simulink model "vehicle_cornering_aero_model"  (R2025b)
settings: Solver=VariableStepAuto  StartTime=0.0  StopTime=100  RelTol=1e-3
model workspace (MAT data in the model file):
  xdot_o = Simulink.Parameter
  xdot_o.Complexity = 'real'
  xdot_o.Dimensions = [1 1]
  xdot_o.DataType = 'auto'
undefined symbols (not defined in the file or in its folder): Ab, Af, brakeBias, cf, Cl, cr, Gamma, gearRatio, hg, Ixx, Kpf, Kpr, l, m, maxPower, maxRev, maxWhlAng, Prs, RCf, RCr, rho, SteerFrq, tireD, track, vref, wd
libraries: simulink_extras x4, simulink x3, vehdynlibtirecommon x3, sharedtransform x3, autolibutils x2, vehdynlibdriver x1, vehdynlibtire x1, autolibshared x1
(part 1 of 2)
settings Model: SimulationMode=accelerator  Creator=keisu  LastModifiedBy=keisu
settings DataIOCC: ReturnWorkspaceOutputs=off

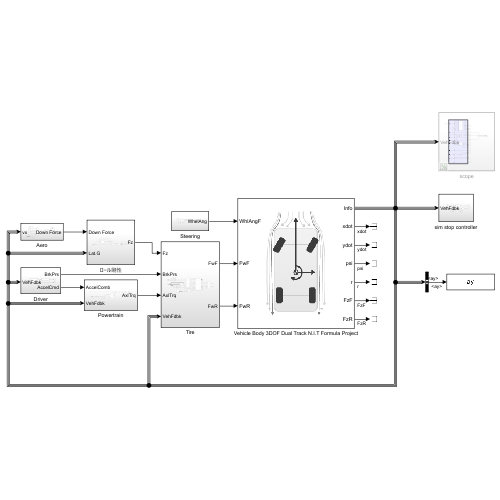
[thumbnail: Simulink's stored preview of the top-level diagram]
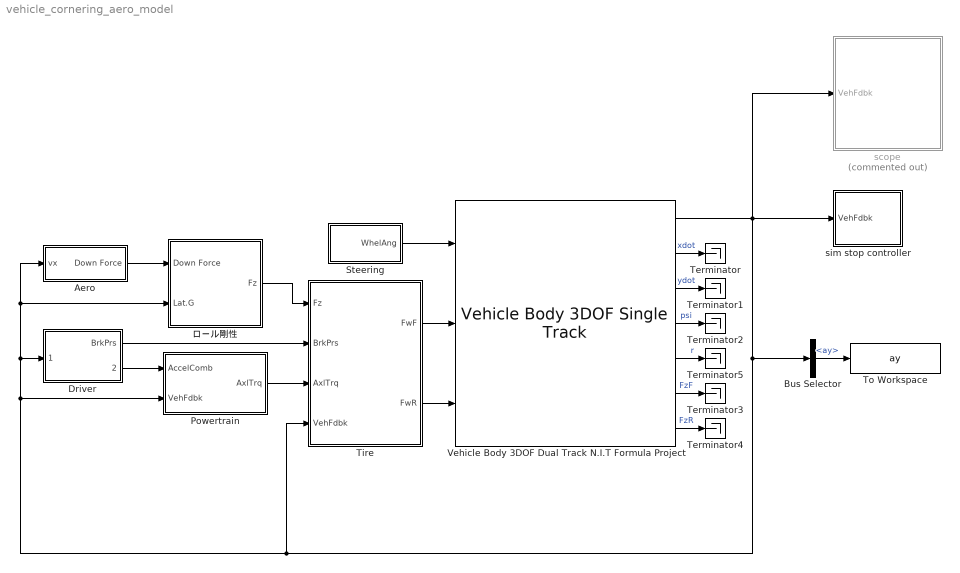
== system vehicle_cornering_aero_model ==
  Aero : Subsystem
  Bus Selector : BusSelector  OutputSignals=BdyFrm.Cg.Acc.ay
  Driver : Subsystem
  Powertrain : Subsystem
  Steering : Subsystem
  Terminator{,1..5} (6 alike) : Terminator
  Tire : Subsystem
  To Workspace : ToWorkspace  VariableName=ay  SaveFormat=Timeseries  SampleTime=-1
  Vehicle Body 3DOF Dual Track N.I.T Formula Project : autolibshared/Vehicle Body 3DOF Single Track  trackMode=Dual  inputMode=External forces  frontSteerMode=on  rearSteerMode=off  windMode=off  muMode=off  extFMode=off  extMMode=off  htchFMode=off  htchMMode=off  extXo=off  extpsio=off  extxdoto=off  extro=off  extYo=off  extTamb=off  extydoto=off  aMode=2  NF=2  NR=2  m=m  a=l*(1-wd)  b=l*wd  h=hg-0.0254*tireD/2  dh=1  hh=0.2  X_o=0  xdot_o=0  CalphaMode=off  sigmaMode=on  d=0  hl=0  w=track  Cy_f=12e3  Cy_r=11e3  sigma_f=.1  sigma_r=.1  alpha_f_brk=[-0.785, -0.628, -0.471, -0.314, -0.157, 0.000, 0.157, 0.314, 0.471, 0.628, 0.785]  Cy_f_data=[2000, 3000, 4000, 5500, 7000, 9000, 7000, 5500, 4000, 3000, 2000]  alpha_r_brk=[-0.785, -0.628, -0.471, -0.314, -0.157, 0.000, 0.157, 0.314, 0.471, 0.628, 0.785]  Cy_r_data=[2000, 3000, 4000, 5500, 7000, 9000, 7000, 5500, 4000, 3000, 2000]  Y_o=0  ydot_o=0  Izz=Izz  psi_o=0  r_o=0  Af=Af  Cd=Cd  Cl=Cl  Cpm=.1  beta_w=[0 0.01:0.01:0.3]  Cs=[0:0.03:0.9]  Cym=[0 1e-6:0.01:0.3]  Pabs=101325  Tair=AirTemp  g=9.81  mu=1  xdot_tol=.01  Fznom=5000  Fxtire_sat=7e4  Fytire_sat=7e4  longOff=0  latOff=0  vertOff=0  wrapAng=off
      settings: LibrarySourceBlock=vehdynlibeom/Vehicle Body 3DOF Dual Track
  scope : Subsystem  Commented=on
  sim stop controller : Subsystem
  ロール剛性 : Subsystem
  wires:
  Vehicle Body 3DOF Dual Track N.I.T Formula Project/1 -> sim stop controller/1(VehFdbk), scope/1(VehFdbk), Bus Selector/1, Aero/1(vx), ロール剛性/2(Lat.G), Driver/1(VehFdbk), Powertrain/2(VehFdbk), Tire/4(VehFdbk)
  Tire/1(FwF) -> Vehicle Body 3DOF Dual Track N.I.T Formula Project/2
  Tire/2(FwR) -> Vehicle Body 3DOF Dual Track N.I.T Formula Project/3
  Vehicle Body 3DOF Dual Track N.I.T Formula Project/2 -> Terminator/1  "xdot"
  Vehicle Body 3DOF Dual Track N.I.T Formula Project/3 -> Terminator1/1  "ydot"
  Vehicle Body 3DOF Dual Track N.I.T Formula Project/4 -> Terminator2/1  "psi"
  Vehicle Body 3DOF Dual Track N.I.T Formula Project/5 -> Terminator5/1  "r"
  Vehicle Body 3DOF Dual Track N.I.T Formula Project/6 -> Terminator3/1  "FzF"
  Vehicle Body 3DOF Dual Track N.I.T Formula Project/7 -> Terminator4/1  "FzR"
  Powertrain/1(AxlTrq) -> Tire/3(AxlTrq)
  ロール剛性/1(Fz) -> Tire/1(Fz)
  Driver/1(BrkPrs) -> Tire/2(BrkPrs)
  Driver/2(AccelCmd) -> Powertrain/1(AccelComb)
  Steering/1(WhelAng) -> Vehicle Body 3DOF Dual Track N.I.T Formula Project/1
  Bus Selector/1 -> To Workspace/1  "<ay>"
  Aero/1(Down Force) -> ロール剛性/1(Down Force)

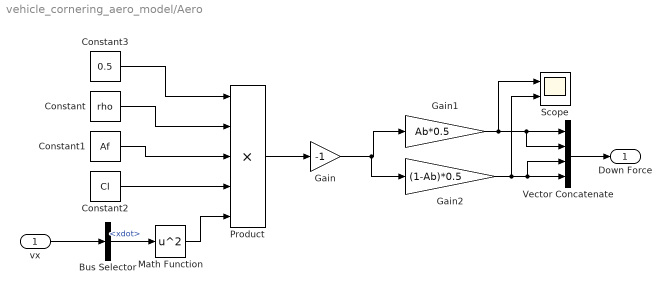
== system vehicle_cornering_aero_model/Aero ==
  vx : Inport
  Bus Selector : BusSelector  OutputSignals=BdyFrm.Cg.Vel.xdot
  Constant : Constant  Value=rho
  Constant1 : Constant  Value=Af
  Constant2 : Constant  Value=Cl
  Constant3 : Constant  Value=0.5
  Gain : Gain  Gain=-1
  Gain1 : Gain  Gain=Ab*0.5
  Gain2 : Gain  Gain=(1-Ab)*0.5
  Math Function : Math  Operator=square
  Product : Product  Inputs=5
  Scope : Scope  NumInputPorts=2
      settings: ActiveDisplayYMinimum=-1  ActiveDisplayYMaximum=1  DataLoggingVariableName=ScopeData2
  Vector Concatenate : Concatenate  NumInputs=4
  Down Force : Outport
  wires:
  vx/1 -> Bus Selector/1
  Constant3/1 -> Product/1
  Constant/1 -> Product/2
  Constant1/1 -> Product/3
  Constant2/1 -> Product/4
  Bus Selector/1 -> Math Function/1  "<xdot>"
  Math Function/1 -> Product/5
  Product/1 -> Gain/1
  Vector Concatenate/1 -> Down Force/1
  Gain/1 -> Gain2/1, Gain1/1
  Gain1/1 -> Scope/1, Vector Concatenate/2, Vector Concatenate/1
  Gain2/1 -> Vector Concatenate/4, Vector Concatenate/3, Scope/2

== system vehicle_cornering_aero_model/Driver ==
  VehFdbk : Inport
  Brake Hydraulics : Subsystem
  Driver : Subsystem
  BrkPrs : Outport
  AccelCmd : Outport  Port=2
  wires:
  Driver/1(DecelCmd) -> Brake Hydraulics/1(BrkPrsCmd)
  Driver/2(AccelCmd) -> AccelCmd/1
  Brake Hydraulics/1(BrkPrs) -> BrkPrs/1
  VehFdbk/1 -> Driver/1(VehFdbk)

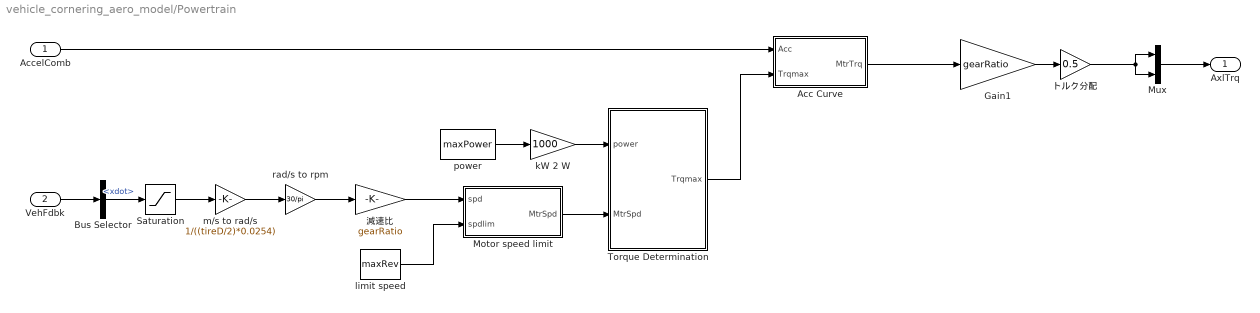
== system vehicle_cornering_aero_model/Powertrain ==
  AccelComb : Inport
  VehFdbk : Inport  Port=2
  Acc Curve : MATLAB Function  TreatAsAtomicUnit=on
  Bus Selector : BusSelector  OutputSignals=BdyFrm.Cg.Vel.xdot
  Gain1 : Gain  Gain=gearRatio
  Motor speed limit : MATLAB Function  TreatAsAtomicUnit=on
  Mux : Mux  Inputs=2
  Saturation : Saturate  UpperLimit=inf  LowerLimit=0
  Torque Determination : MATLAB Function  TreatAsAtomicUnit=on
  kW 2 W : Gain  Gain=1000
  limit speed : Constant  Value=maxRev
  m/s to rad/s : Gain  Gain=1/((tireD/2)*0.0254)
  power : Constant  Value=maxPower
  rad/s to rpm : Gain  Gain=30/pi
  トルク分配 : Gain  Gain=0.5
  減速比 : Gain  Gain=gearRatio
  AxlTrq : Outport
  wires:
  power/1 -> kW 2 W/1
  limit speed/1 -> Motor speed limit/2(spdlim)
  rad/s to rpm/1 -> 減速比/1
  Torque Determination/1(Trqmax) -> Acc Curve/2(Trqmax)
  AccelComb/1 -> Acc Curve/1(Acc)
  減速比/1 -> Motor speed limit/1(spd)
  m/s to rad/s/1 -> rad/s to rpm/1
  kW 2 W/1 -> Torque Determination/1(power)
  Motor speed limit/1(MtrSpd) -> Torque Determination/2(MtrSpd)
  Saturation/1 -> m/s to rad/s/1
  VehFdbk/1 -> Bus Selector/1
  Gain1/1 -> トルク分配/1
  Mux/1 -> AxlTrq/1
  Acc Curve/1(MtrTrq) -> Gain1/1
  Bus Selector/1 -> Saturation/1  "<xdot>"
  トルク分配/1 -> Mux/2, Mux/1

== system vehicle_cornering_aero_model/Steering ==
  <1 : Saturate  UpperLimit=1  LowerLimit=-1
  Degrees to Radians2 : simulink_extras/Transformations/Degrees to Radians
  Dot Product : DotProduct  OutDataTypeStr=Inherit: Inherit via internal rule
  Vector Concatenate : Concatenate
  最大ホール端転舵角 : Constant  Value=maxWhlAng
  転舵周波数 : simulink/Sources/Ramp  slope=1/SteerFrq  start=steerstartTime  InitialOutput=0
  WhelAng : Outport
  wires:
  転舵周波数/1 -> <1/1
  Dot Product/1 -> Degrees to Radians2/1
  <1/1 -> Dot Product/2
  最大ホール端転舵角/1 -> Dot Product/1
  Degrees to Radians2/1 -> Vector Concatenate/2, Vector Concatenate/1
  Vector Concatenate/1 -> WhelAng/1

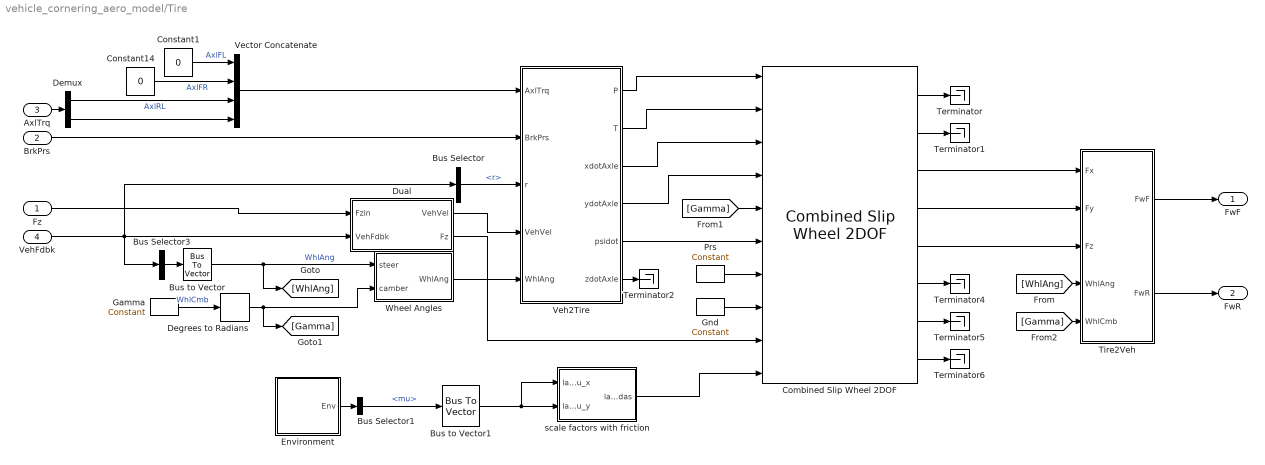
== system vehicle_cornering_aero_model/Tire ==
  Fz : Inport
  BrkPrs : Inport  Port=2
  AxlTrq : Inport  Port=3
  VehFdbk : Inport  Port=4
  Bus Selector : BusSelector  OutputSignals=BdyFrm.Cg.AngVel.r
  Bus Selector1 : BusSelector  OutputSignals=Gnd.mu
  Bus Selector3 : BusSelector  OutputSignals=BdyFrm.FrntAxl.Steer.WhlAngFL,BdyFrm.FrntAxl.Steer.WhlAngFR,BdyFrm.RearAxl.Steer.WhlAngRL,BdyFrm.RearAxl.Steer.WhlAngRR  OutputAsBus=on
  Bus to Vector : BusToVector
  Bus to Vector1 : BusToVector
  Combined Slip Wheel 2DOF : vehdynlibtire/Combined Slip Wheel 2DOF  tireType=External file  tireParamSet=TIRfile  vertType=Magic Formula  plySteer=off  turnslip=off  BrakeType=Disc  mu_static=mu_static  mu_kinetic=mu_kinetic  drum_abore=0.0508  drum_a=0.123  drum_c=0.212  drum_r=0.15  drum_theta1=0  drum_theta2=126  disk_abore=disk_abore  Rm=Rm  num_pads=num_pads  brake_p_bpt=[1 11.4736842105263 21.9473684210526 32.4210526315789 42.8947368421053 53.3684210526316 63.8421052631579 74.3157894736842 84.7894736842105 95.2631578947368 105.736842105263 116.210526315789 126.684210526316 137.157894736842 147.631578947368 158.105263157895 168.578947368421 179.052631578947 189.526315789474 200]  brake_n_bpt=[0 52.6315789473684 105.263157894737 157.894736842105 210.526315789474 263.157894736842 315.789473684211 368.421052631579 421.052631578947 473.684210526316 526.315789473684 578.947368421053 631.578947368421 684.210526315789 736.842105263158 789.473684210526 842.105263157895 894.736842105263 947.368421052632 1000]  f_brake_t=[43.4900602404453 42.5056030554862 41.5350898940194 40.5780454442085 39.6340111501808 38.7025443887544 37.7832176914519 36.8756180088306 35.9793460143796 35.0940154454303 34.2192524787115 33.3546951383474 32.4999927342521 31.6548053290159 30.8188032315107 29.991666515561 29.1730845621415 28.362755623661 27.5603864089927 26.765691687993;498.991217495636 487.695866636631 476.560505099801 465.579679307235 454.748127933653 444.060772460445 433.51270824929 423.099196101319 412.81565427025 402.657650900201 392.620896861006 382.701238955775 372.894653477208 363.197240090814 353.605216024701 344.114910546964 334.722759712992 325.425301366216 316.219170376863 307.10109410434;954.492374750826 932.886130217776 911.585920305583 890.581313170261 869.862244717126 849.419000532136 829.242198807128 809.322774193808 789.651962526121 770.221286354971 751.0225412433 732.047782773203 713.289314220164 694.739674852612 676.391628817892 658.238154578366 640.272434863842 622.48784710877 604.877954344734 587.436496520688;1409.99353200602 1378.07639379892 1346.61133551136 1315.58294703329 1284.9763615006 1254.77722860383 1224.97168936497 1195.5463522863 1166.48827078199 1137.78492180974 1109.42418562559 1081.39432659063 1053.68397496312 1026.28210961441 999.178041611083 972.361398609768 945.822110014692 919.550392851325 893.536738312604 867.771898937035;1865.49468926121 1823.26665738007 1781.63675071715 1740.58458089631 1700.09047828407 1660.13545667552 1620.7011799228 1581.76993037878 1543.32457903786 1505.34855726451 1467.82583000789 1430.74087040806 1394.07863570608 1357.82454437621 1321.96445440427 1286.48464264117 1251.37178516554 1216.61293859388 1182.19552228048 1148.10730135338;2320.9958465164 2268.45692096121 2216.66216592293 2165.58621475934 2115.20459506754 2065.49368474721 2016.43067048064 1967.99350847127 1920.16088729373 1872.91219271928 1826.22747439018 1780.08741422549 1734.47329644903 1689.36697913801 1644.75086719747 1600.60788667257 1556.92146031639 1513.67548433643 1470.85430624835 1428.44270376973;2776.49700377159 2713.64718454235 2651.68758112871 2590.58784862237 2530.31871185102 2470.8519128189 2412.16016103848 2354.21708656376 2296.9971955496 2240.47582817405 2184.62911877248 2129.43395804292 2074.86795719199 2020.9094138998 1967.53727999066 1914.73113070398 1862.47113546724 1810.73803007899 1759.51309021622 1708.77810618608;3231.99816102678 3158.8374481235 3086.71299633449 3015.58948248539 2945.43282863449 2876.21014089059 2807.88965159632 2740.44066465625 2673.83350380547 2608.03946362882 2543.03076315477 2478.78050186034 2415.26261793494 2352.4518486616 2290.32369278385 2228.85437473538 2168.02081061809 2107.80057582154 2048.17187418409 1989.11350860242;3687.49931828197 3604.02771170464 3521.73841154027 3440.59111634842 3360.54694541796 3281.56836896228 3203.61914215416 3126.66424274874 3050.66981206134 2975.60309908359 2901.43240753707 2828.12704567777 2755.6572786779 2683.9942834234 2613.11010557704 2542.97761876678 2473.57048576894 2404.8631215641 2336.83065815196 2269.44891101877;4143.00047553716 4049.21797528579 3956.76382674606 3865.59275021144 3775.66106220143 3686.92659703397 3599.34863271199 3512.88782084123 3427.50612031721 3343.16673453836 3259.83405191936 3177.4735894952 3096.05193942085 3015.5367181852 2935.89651837023 2857.10086279818 2779.12016091979 2701.92566730665 2625.48944211983 2549.78431343512;4598.50163279235 4494.40823886693 4391.78924195184 4290.59438407447 4190.77517898491 4092.28482510566 3995.07812326983 3899.11139893372 3804.34242857308 3710.73036999313 3618.23569630166 3526.82013331263 3436.44660016381 3347.079152947 3258.68293116342 3171.22410682959 3084.66983607064 2998.98821304921 2914.1482260877 2830.11971585147;5054.00279004754 4939.59850244808 4826.81465715762 4715.59601793749 4605.88929576838 4497.64305317735 4390.80761382767 4285.3349770262 4181.17873682896 4078.2940054479 3976.63734068395 3876.16667713006 3776.84126090677 3678.62158770879 3581.46934395661 3485.34735086099 ...(+2764 chars)]  NOMPRES=100000  PRESMAX=99780  PRESMIN=45540  FNOMIN=1500  FZMAX=1688  FZMIN=185  VXLOW=1  KPUMAX=1.5  KPUMIN=-1.5  ALPMAX=0.2338  ALPMIN=-0.2293  CAMMAX=0.0699  CAMMIN=-0.0699  LONGVL=10  FxRelFreqLwrLim=200*pi  FyRelFreqLwrLim=200*pi  MyRelFreqLwrLim=100*pi  omegao=0  UNLOADED_RADIUS=0.2667  WIDTH=0.2032  RIM_RADIUS=0.1651  ASPECT_RATIO=0.5  MASS=9.3  IYY=0.736  br=1e-3  GRAVITY=-9.81  zo=0  zdoto=0  BREFF=13.804  DREFF=1.08343  FREFF=0.16356  Q_RE0=0.9974  Q_V1=0.00077  Q_V2=9e-05  Q_FZ1=0  Q_FZ2=482.2  Q_FZ3=0  Q_FCX=0  Q_FCY=0  Q_FCY2=0  PFZ1=0.7098  VERTICAL_STIFFNESS=142605.8  VERTICAL_DAMPING=50  BOTTOM_OFFST=0.01  BOTTOM_STIFF=2000000  Q_CAM1=0  Q_CAM2=0  Q_CAM3=0  Q_FYS1=0  Q_FYS2=0  Q_FYS3=0  LONGITUDINAL_STIFFNESS=256665.8  LATERAL_STIFFNESS=128332.9  PCFX1=0.17504  PCFX2=0  PCFX3=0  PCFY1=-0.03642  PCFY2=-0.27821  PCFY3=0.85328  Q_RA1=0.671  Q_RA2=0.733  Q_RB1=1.059  Q_RB2=-1.1878  PCX1=1.6115  PDX1=2.2174  PDX2=-3.7188e-11  PDX3=6.2143  PEX1=-3.9492e-12  PEX2=-0.45667  PEX3=-0.6  PEX4=0.9  PKX1=26.7995  PKX2=21.0631  PKX3=-1.4239  PHX1=0.00082836  PHX2=0.0023285  PVX1=-0.049942  PVX2=-0.1  PPX1=-2.2632  PPX2=-2.7144  PPX3=-0.22349  PPX4=0.31229  RBX1=14.591  RBX2=8.7174  RBX3=230.1041  RCX1=1.0245  REX1=0.94083  REX2=1  RHX1=0.0017088  QSX1=0  QSX2=1.5  QSX3=0.1  QSX4=0.1  QSX5=0  QSX6=0  QSX7=0.1  QSX8=0  QSX9=0  QSX10=0  QSX11=0  QSX12=0  QSX13=0  QSX14=0  PPMX1=0  PCY1=1.5  PDY1=2.4125  PDY2=-0.5  PDY3=8.211  PEY1=1.0849  PEY2=0.34897  PEY3=-0.44519  PEY4=2.8269  PEY5=-47.8511  PKY1=-21.771  PKY2=0.87137  PKY3=1  PKY4=2  PKY5=13.311  PKY6=-1.0665  PKY7=0.89924  PHY1=-0.00067702  PHY2=0.00021021  PVY1=-0.057811  PVY2=0.17638  PVY3=-0.1609  PVY4=-3.0413  PPY1=0.44211  PPY2=1.2522  PPY3=-0.25468  PPY4=-0.081179  PPY5=0.56704  RBY1=39.9961  RBY2=40  RBY3=0.070501  RBY4=-89.9999  RCY1=0.96955  REY1=0.9432  REY2=0.53891  RHY1=0.018118  RHY2=0.024952  RVY1=0  RVY2=0  RVY3=0  RVY4=0  RVY5=0  RVY6=0  QSY1=0  QSY2=0  QSY3=0  QSY4=0  QSY5=0  QSY6=0  QSY7=0  QSY8=0  QBZ1=2.2204e-16  QBZ2=0  QBZ3=0  QBZ4=0  QBZ5=0  QBZ6=0  QBZ9=0  QBZ10=0  QCZ1=0.1  QDZ1=0.1  QDZ2=0  QDZ3=0  QDZ4=0  QDZ6=0  QDZ7=0  QDZ8=0  QDZ9=0  QDZ10=0  QDZ11=0  QEZ1=0  QEZ2=0  QEZ3=0  QEZ4=0  QEZ5=0  QHZ1=0  QHZ2=0  QHZ3=0  QHZ4=0  PPZ1=0  PPZ2=0  SSZ1=0  SSZ2=0  SSZ3=0  SSZ4=0  PDXP1=0  PDXP2=0  PDXP3=0  PKYP1=0  PDYP1=0  PDYP2=0  PDYP3=0  PDYP4=0  PHYP1=0  PHYP2=0  PHYP3=0  PHYP4=0  PECP1=0  PECP2=0  QDTP1=0  QCRP1=0  QCRP2=0  QBRP1=0  QDRP1=0  QDRP2=0  aMode=2
  Constant1 : Constant  Value=0
  Constant14 : Constant  Value=0
  Degrees to Radians : simulink_extras/Transformations/Degrees to Radians
  Demux : Demux  Outputs=2
  Dual : Subsystem  VariantControl=1
  Environment : Subsystem
      mask Display: disp('Environment')
  Gamma : vehdynlibtirecommon/Constant  const=Gamma  numWheels=4
  Gnd : vehdynlibtirecommon/Constant  const=0  numWheels=4
  Prs : vehdynlibtirecommon/Constant  const=Prs  numWheels=4
  Terminator{,1..2,4..6} (6 alike) : Terminator
  Tire2Veh : Subsystem
  Vector Concatenate : Concatenate  NumInputs=4
  Veh2Tire : Subsystem
  Wheel Angles : Subsystem
  scale factors with friction : Subsystem  mask{numWheels=4}
      mask prompts: numWheels "Number of wheels"
  FwF : Outport
  FwR : Outport  Port=2
  wires:
  [WhlAng] -> Tire2Veh/4(WhlAng)
  Gamma/1 -> Degrees to Radians/1  "WhlCmb"
  Bus Selector/1 -> Veh2Tire/3(r)  "<r>"
  VehFdbk/1 -> Bus Selector/1, Bus Selector3/1, Dual/2(VehFdbk)
  Dual/1(VehVel) -> Veh2Tire/4(VehVel)
  Dual/2(Fz) -> Combined Slip Wheel 2DOF/9
  Wheel Angles/1(WhlAng) -> Veh2Tire/5(WhlAng)
  Bus to Vector/1 -> [WhlAng], Wheel Angles/1(steer)  "WhlAng"
  Veh2Tire/6(zdotAxle) -> Terminator2/1
  Combined Slip Wheel 2DOF/4 -> Tire2Veh/2(Fy)
  Combined Slip Wheel 2DOF/7 -> Terminator5/1
  Combined Slip Wheel 2DOF/3 -> Tire2Veh/1(Fx)
  Veh2Tire/3(xdotAxle) -> Combined Slip Wheel 2DOF/3
  Gnd/1 -> Combined Slip Wheel 2DOF/8
  Veh2Tire/1(P) -> Combined Slip Wheel 2DOF/1
  Combined Slip Wheel 2DOF/8 -> Terminator6/1
  [Gamma] -> Combined Slip Wheel 2DOF/5
  Combined Slip Wheel 2DOF/6 -> Terminator4/1
  Veh2Tire/5(psidot) -> Combined Slip Wheel 2DOF/6
  Combined Slip Wheel 2DOF/1 -> Terminator/1
  Combined Slip Wheel 2DOF/5 -> Tire2Veh/3(Fz)
  Prs/1 -> Combined Slip Wheel 2DOF/7
  [Gamma] -> Tire2Veh/5(WhlCmb)
  Veh2Tire/4(ydotAxle) -> Combined Slip Wheel 2DOF/4
  Veh2Tire/2(T) -> Combined Slip Wheel 2DOF/2
  Combined Slip Wheel 2DOF/2 -> Terminator1/1
  Tire2Veh/1(FwF) -> FwF/1
  Bus Selector3/1 -> Bus to Vector/1
  Vector Concatenate/1 -> Veh2Tire/1(AxlTrq)
  Tire2Veh/2(FwR) -> FwR/1
  Bus Selector1/1 -> Bus to Vector1/1  "<mu>"
  Environment/1(Env) -> Bus Selector1/1
  Bus to Vector1/1 -> scale factors with friction/1(lamda_mu_x), scale factors with friction/2(lamda_mu_y)
  Degrees to Radians/1 -> [Gamma], Wheel Angles/2(camber)
  scale factors with friction/1(lambdas) -> Combined Slip Wheel 2DOF/10
  AxlTrq/1 -> Demux/1
  Demux/2 -> Vector Concatenate/4
  Demux/1 -> Vector Concatenate/3  "AxlRL"
  BrkPrs/1 -> Veh2Tire/2(BrkPrs)
  Constant14/1 -> Vector Concatenate/2  "AxlFR"
  Constant1/1 -> Vector Concatenate/1  "AxlFL"
  Fz/1 -> Dual/1(Fzin)

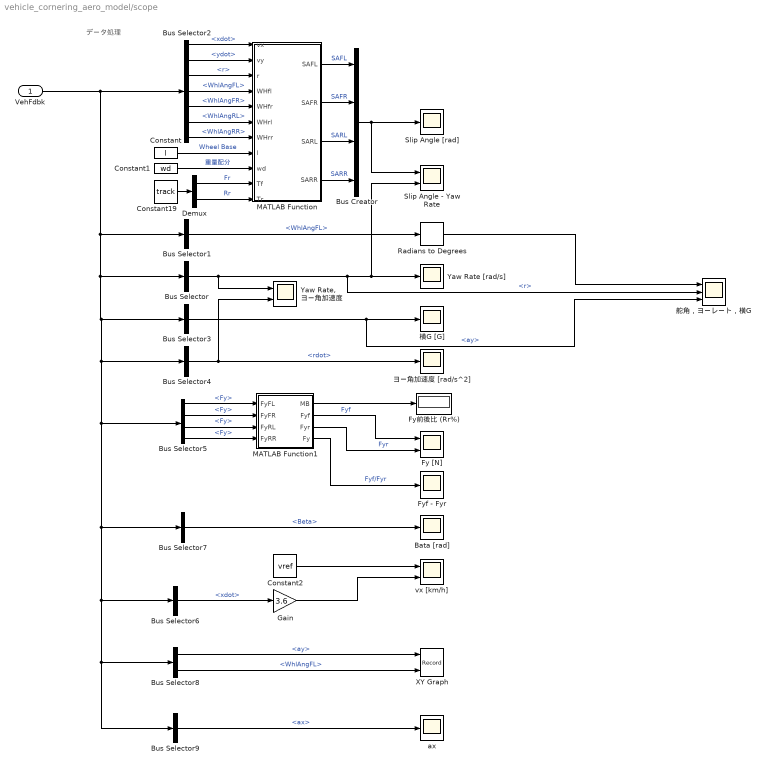
== system vehicle_cornering_aero_model/scope ==
  note: データ処理
  VehFdbk : Inport
  Bata [rad] : Scope
      settings: ActiveDisplayYMinimum=-1  ActiveDisplayYMaximum=1  DataLoggingVariableName=ScopeData24
  Bus Creator : BusCreator  Inputs=4
  Bus Selector : BusSelector  OutputSignals=BdyFrm.Cg.AngVel.r
  Bus Selector1 : BusSelector  OutputSignals=BdyFrm.FrntAxl.Steer.WhlAngFL
  Bus Selector2 : BusSelector  OutputSignals=BdyFrm.Cg.Vel.xdot,BdyFrm.Cg.Vel.ydot,BdyFrm.Cg.AngVel.r,BdyFrm.FrntAxl.Steer.WhlAngFL,BdyFrm.FrntAxl.Steer.WhlAngFR,BdyFrm.RearAxl.Steer.WhlAngRL,BdyFrm.RearAxl.Steer.WhlAngRR
  Bus Selector3 : BusSelector  OutputSignals=BdyFrm.Cg.Acc.ay
  Bus Selector4 : BusSelector  OutputSignals=BdyFrm.Cg.AngAcc.rdot
  Bus Selector5 : BusSelector  OutputSignals=BdyFrm.Forces.FrntAxl.Lft.Fy,BdyFrm.Forces.FrntAxl.Rght.Fy,BdyFrm.Forces.RearAxl.Lft.Fy,BdyFrm.Forces.RearAxl.Rght.Fy
  Bus Selector6 : BusSelector  OutputSignals=BdyFrm.Cg.Vel.xdot
  Bus Selector7 : BusSelector  OutputSignals=BdyFrm.Cg.Ang.Beta
  Bus Selector8 : BusSelector  OutputSignals=BdyFrm.Cg.Acc.ay,BdyFrm.FrntAxl.Steer.WhlAngFL
  Bus Selector9 : BusSelector  OutputSignals=BdyFrm.Cg.Acc.ax
  Constant : Constant  Value=l
  Constant1 : Constant  Value=wd
  Constant19 : Constant  Value=track
  Constant2 : Constant  Value=vref
  Demux : Demux  Outputs=2
  Fy [N] : Scope  NumInputPorts=2
      settings: ActiveDisplayYMinimum=-332.96990553585255  ActiveDisplayYMaximum=3062.84620162171  DataLoggingVariableName=ScopeData25
  Fyf - Fyr : Scope
      settings: ActiveDisplayYMinimum=-1174.9727661514175  ActiveDisplayYMaximum=10574.754895362483  DataLoggingVariableName=ScopeData21
  Fy前後比 (Rr%) : Display
  Gain : Gain  Gain=3.6
  MATLAB Function : MATLAB Function  TreatAsAtomicUnit=on
  MATLAB Function1 : MATLAB Function  TreatAsAtomicUnit=on
  Radians to Degrees : simulink_extras/Transformations/Radians to Degrees
  Slip Angle - Yaw Rate : Scope  NumInputPorts=2
      settings: ActiveDisplayYMinimum=-0.74882572671582448  ActiveDisplayYMaximum=1.1744319785697512  DataLoggingVariableName=ScopeData26
  Slip Angle [rad] : Scope
      settings: ActiveDisplayYMinimum=-0.384467573960002  ActiveDisplayYMaximum=0.088617945349714261  DataLoggingVariableName=ScopeData14
  XY Graph : Record  NumPorts=2.0  FileSettingsInternal="{\"entries\":[{\"content\":{\"excelSettings\":{\"content\":{},\"type\":\"Streamout.ExcelSettings\"},\"parquetSettings\":{\"content\":{},\"type\":\"Streamout.ParquetSettings\"}},\"type\":\"Streamout.FileSettingStorage\",\"uuid\":\"\"}],\"packageUris\":[\"http:\\/\\/schema.mathworks.com\\/mf0\\/streamout_blocks\\/R2020a\"],\"version\":\"1.0\"}"  FrameSettings=[0, 0]  Layout=[1 1]  SignalsInternal="{\"entries\":[{\"content\":{\"signals\":[{\"content\":{\"blockPath\":[],\"dimensions\":[1],\"domain\":\"\",\"lineColor\":\"#64d413\",\"lineWidth\":2,\"port\":1,\"signalID\":1,\"signalName\":\"<ay>\"},\"type\":\"RecordBlkView.Signal\",\"uuid\":\"\"},{\"content\":{\"blockPath\":[],\"dimensions\":[1],\"domain\":\"\",\"lineColor\":\"#ff13a6\",\"lineWidth\":2,\"port\":2,\"signalID\":2,\"signalName\":\"<WhlAngFL>\"},\"type\":\"RecordBlkView.Signal\",\"uuid\":\"\"}]},\"type\":\"RecordBlkView.InputSignals\",\"uuid\":\"\"}],\"packageUris\":[\"http:\\/\\/schema.mathworks.com\\/mf0\\/streamout_blocks\\/R2020a\"],\"version\":\"1.0\"}"  VisualizationBindings="{\"xyplotplugin\":{\"info\":[{\"series\":[],\"subplotID\":1}]}}"  CompatibilityTag=XY
  Yaw Rate [rad/s] : Scope
      settings: ActiveDisplayYMinimum=-0.62750669087428634  ActiveDisplayYMaximum=5.6475602178685378  DataLoggingVariableName=ScopeData18
  "Yaw Rate, ヨー角加速度" : Scope  NumInputPorts=2
      settings: ActiveDisplayYMinimum=-1.3415902700915119  ActiveDisplayYMaximum=11.600558391109077  DataLoggingVariableName=ScopeData23
  ax : Scope
      settings: ActiveDisplayYMinimum=-1  ActiveDisplayYMaximum=1  DataLoggingVariableName=ScopeData29
  vx [km/h] : Scope  NumInputPorts=2
      settings: ActiveDisplayYMinimum=-7.5588295902982621  ActiveDisplayYMaximum=68.029466312684377  DataLoggingVariableName=ScopeData20
  ヨー角加速度 [rad/s^2] : Scope
      settings: ActiveDisplayYMinimum=-46.370009425393938  ActiveDisplayYMaximum=30.296576057409077  DataLoggingVariableName=ScopeData22
  横G [G] : Scope
      settings: ActiveDisplayYMinimum=-0.14914054039878477  ActiveDisplayYMaximum=1.3422648508032233  DataLoggingVariableName=ScopeData19
  舵角，ヨーレート，横G : Scope  NumInputPorts=3
      settings: ActiveDisplayYMinimum=-0.259247770248695  ActiveDisplayYMaximum=2.3332299322382557  DataLoggingVariableName=ScopeData27
  wires:
  Bus Creator/1 -> Slip Angle [rad]/1, Slip Angle - Yaw Rate/1
  Bus Selector1/1 -> Radians to Degrees/1  "<WhlAngFL>"
  VehFdbk/1 -> Bus Selector7/1, Bus Selector9/1, Bus Selector8/1, Bus Selector6/1, Bus Selector5/1, Bus Selector4/1, Bus Selector3/1, Bus Selector/1, Bus Selector1/1, Bus Selector2/1
  Bus Selector2/5 -> MATLAB Function/5(WHfr)  "<WhlAngFR>"
  MATLAB Function/3(SARL) -> Bus Creator/3  "SARL"
  MATLAB Function/1(SAFL) -> Bus Creator/1  "SAFL"
  Bus Selector2/4 -> MATLAB Function/4(WHfl)  "<WhlAngFL>"
  Bus Selector2/1 -> MATLAB Function/1(vx)  "<xdot>"
  Demux/1 -> MATLAB Function/10(Tf)  "Fr"
  Constant1/1 -> MATLAB Function/9(wd)  "重量配分"
  Bus Selector2/3 -> MATLAB Function/3(r)  "<r>"
  MATLAB Function/2(SAFR) -> Bus Creator/2  "SAFR"
  Demux/2 -> MATLAB Function/11(Tr)  "Rr"
  MATLAB Function/4(SARR) -> Bus Creator/4  "SARR"
  Bus Selector2/6 -> MATLAB Function/6(WHrl)  "<WhlAngRL>"
  Bus Selector2/7 -> MATLAB Function/7(WHrr)  "<WhlAngRR>"
  Constant19/1 -> Demux/1
  Constant/1 -> MATLAB Function/8(l)  "Wheel Base"
  Bus Selector2/2 -> MATLAB Function/2(vy)  "<ydot>"
  Bus Selector/1 -> 舵角，ヨーレート，横G/2, Yaw Rate [rad/s]/1, Slip Angle - Yaw Rate/2, "Yaw Rate, ヨー角加速度"/1  "<r>"
  Bus Selector3/1 -> 舵角，ヨーレート，横G/3, 横G [G]/1  "<ay>"
  Bus Selector4/1 -> ヨー角加速度 [rad/s^2]/1, "Yaw Rate, ヨー角加速度"/2  "<rdot>"
  Bus Selector5/1 -> MATLAB Function1/1(FyFL)  "<Fy>"
  Bus Selector5/2 -> MATLAB Function1/2(FyFR)  "<Fy>"
  Bus Selector5/3 -> MATLAB Function1/3(FyRL)  "<Fy>"
  Bus Selector5/4 -> MATLAB Function1/4(FyRR)  "<Fy>"
  MATLAB Function1/1(MB) -> Fy前後比 (Rr%)/1
  MATLAB Function1/2(Fyf) -> Fy [N]/1  "Fyf"
  MATLAB Function1/3(Fyr) -> Fy [N]/2  "Fyr"
  Bus Selector6/1 -> Gain/1  "<xdot>"
  Gain/1 -> vx [km/h]/2
  Constant2/1 -> vx [km/h]/1
  MATLAB Function1/4(Fy) -> Fyf - Fyr/1  "Fyf/Fyr"
  Bus Selector7/1 -> Bata [rad]/1  "<Beta>"
  Bus Selector8/1 -> XY Graph/1  "<ay>"
  Bus Selector8/2 -> XY Graph/2  "<WhlAngFL>"
  Bus Selector9/1 -> ax/1  "<ax>"
  Radians to Degrees/1 -> 舵角，ヨーレート，横G/1

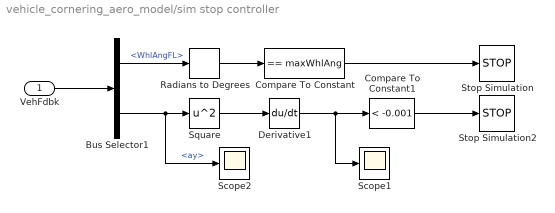
== system vehicle_cornering_aero_model/sim stop controller ==
  VehFdbk : Inport
  Bus Selector1 : BusSelector  OutputSignals=BdyFrm.FrntAxl.Steer.WhlAngFL,BdyFrm.Cg.Acc.ay
  Compare To Constant : simulink/Logic and Bit Operations/Compare To Constant  relop===  const=maxWhlAng  OutDataTypeStr=boolean
  Compare To Constant1 : simulink/Logic and Bit Operations/Compare To Constant  relop=<  const=-0.001  OutDataTypeStr=boolean
  Derivative1 : Derivative
  Radians to Degrees : simulink_extras/Transformations/Radians to Degrees
  Scope1 : Scope
      settings: ActiveDisplayYMinimum=-0.0002535772325386222  ActiveDisplayYMaximum=0.0022821950928476  DataLoggingVariableName=ScopeData3
  Scope2 : Scope
      settings: ActiveDisplayYMinimum=-0.025196586189438902  ActiveDisplayYMaximum=0.22676927570494698  DataLoggingVariableName=ScopeData4
  Square : Math  Operator=square
  Stop Simulation : Stop
  Stop Simulation2 : Stop
  wires:
  Compare To Constant/1 -> Stop Simulation/1
  Radians to Degrees/1 -> Compare To Constant/1
  VehFdbk/1 -> Bus Selector1/1
  Bus Selector1/1 -> Radians to Degrees/1  "<WhlAngFL>"
  Bus Selector1/2 -> Square/1, Scope2/1  "<ay>"
  Derivative1/1 -> Scope1/1, Compare To Constant1/1
  Compare To Constant1/1 -> Stop Simulation2/1
  Square/1 -> Derivative1/1

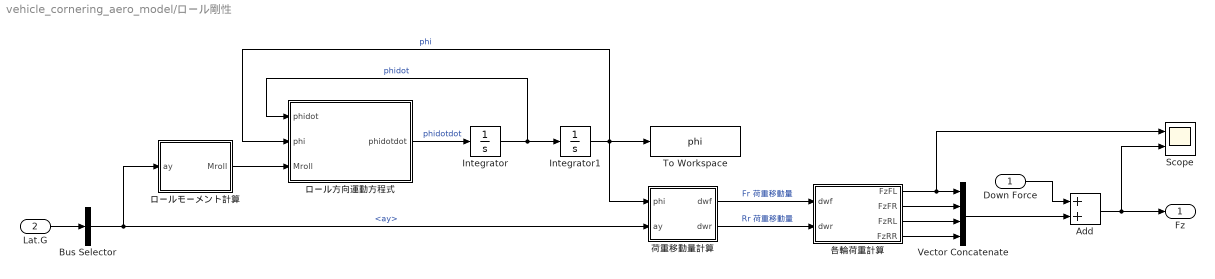
== system vehicle_cornering_aero_model/ロール剛性 ==
  Down Force : Inport
  Lat.G : Inport  Port=2
  Add : Sum
  Bus Selector : BusSelector  OutputSignals=BdyFrm.Cg.Acc.ay
  Integrator : Integrator
  Integrator1 : Integrator
  Scope : Scope  NumInputPorts=2
      settings: ActiveDisplayYMinimum=-11.525534753656018  ActiveDisplayYMaximum=1574.5496108637544
  To Workspace : ToWorkspace  VariableName=phi  SaveFormat=Timeseries  SampleTime=-1
  Vector Concatenate : Concatenate  NumInputs=4
  ロールモーメント計算 : MATLAB Function  TreatAsAtomicUnit=on
  ロール方向運動方程式 : MATLAB Function  TreatAsAtomicUnit=on
  各輪荷重計算 : MATLAB Function  TreatAsAtomicUnit=on
  荷重移動量計算 : MATLAB Function  TreatAsAtomicUnit=on
  Fz : Outport
  wires:
  Lat.G/1 -> Bus Selector/1
  Bus Selector/1 -> ロールモーメント計算/1(ay), 荷重移動量計算/2(ay)  "<ay>"
  荷重移動量計算/2(dwr) -> 各輪荷重計算/2(dwr)  "Rr 荷重移動量"
  荷重移動量計算/1(dwf) -> 各輪荷重計算/1(dwf)  "Fr 荷重移動量"
  各輪荷重計算/1(FzFL) -> Scope/1, Vector Concatenate/1
  各輪荷重計算/2(FzFR) -> Vector Concatenate/2
  各輪荷重計算/3(FzRL) -> Vector Concatenate/3
  各輪荷重計算/4(FzRR) -> Vector Concatenate/4
  ロールモーメント計算/1(Mroll) -> ロール方向運動方程式/3(Mroll)
  ロール方向運動方程式/1(phidotdot) -> Integrator/1  "phidotdot"
  Integrator/1 -> Integrator1/1, ロール方向運動方程式/1(phidot)  "phidot"
  Integrator1/1 -> To Workspace/1, ロール方向運動方程式/2(phi), 荷重移動量計算/1(phi)  "phi"
  Vector Concatenate/1 -> Add/2
  Add/1 -> Scope/2, Fz/1
  Down Force/1 -> Add/1

== system vehicle_cornering_aero_model/Driver/Brake Hydraulics ==
  BrkPrsCmd : Inport
  Dead Zone : DeadZone  LowerValue=-inf  UpperValue=1e-3  ZeroCross=off
  Front Bias : Constant
  Gain4 : Gain  Gain=1e6
  Mux : Mux
  Product : Product
  Rear Bias : Constant  Value=brakeBias
  Selector : Selector  InputPortWidth=1  IndexOptions=Index vector (dialog)  Indices=[1 1 1 1]  OutputSizes=1
  Valve : autolibutils/Cont LPF  wc=40*pi  AbsoluteTolerance=auto  aMode=2
  BrkPrs : Outport  VectorParamsAs1DForOutWhenUnconnected=off
  wires:
  BrkPrsCmd/1 -> Valve/1
  Valve/1 -> Dead Zone/1  "Flow"
  Gain4/1 -> BrkPrs/1
  Front Bias/1 -> Mux/2, Mux/1
  Rear Bias/1 -> Mux/3, Mux/4
  Product/1 -> Gain4/1
  Mux/1 -> Product/1
  Selector/1 -> Product/2
  Dead Zone/1 -> Selector/1

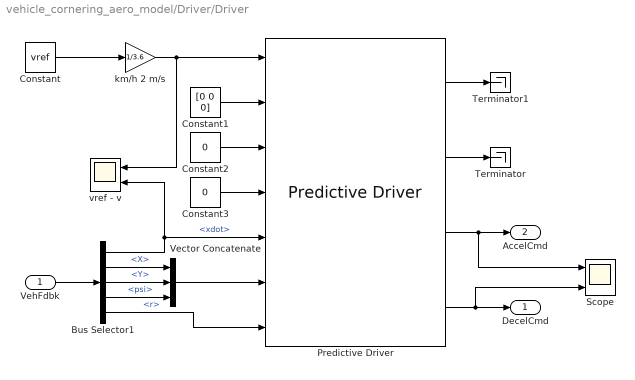
== system vehicle_cornering_aero_model/Driver/Driver ==
  VehFdbk : Inport
  Bus Selector1 : BusSelector  OutputSignals=BdyFrm.Cg.Vel.xdot,InertFrm.Cg.Disp.X,InertFrm.Cg.Disp.Y,InertFrm.Cg.Ang.psi,BdyFrm.Cg.AngVel.r
  Constant : Constant  Value=vref
  Constant1 : Constant  Value=[0 0 0]
  Constant2 : Constant  Value=0
  Constant3 : Constant  Value=0
  Predictive Driver : vehdynlibdriver/Predictive Driver  extAccelOvr=off  extDecelOvr=off  extAccelHld=off  extDecelHld=off  extAccelZero=off  extDecelZero=off  extSteerOvr=off  extSteerHld=off  extSteerZero=off  cntrlType=Predictive  cntrlTypeLat=Stanley  shftType=None  coordMode=SAE J670 (Z-down)  refType=Reference pose  velUnits=m/s  angUnits=rad  gearOut=off  steerOut=off  Kp=10  Ki=5  Kff=.1  Kg=0  VehVelVec=[0 100]  KffVec=[.1 .1]  KpVec=[10 10]  KiVec=[5 5]  KgVec=[0 0]  vnom=5  Kaw=1  tauerr=.01  tau=.1  L=6  Kpt=(70*gearRatio)/(0.0254*tireD/2)  aR=200  bR=2.5  cR=.5  g=9.81  vecPose=on  dynamMode=on  PositionGainF=2.5  PositionGainR=.5  YawRateGain=.1  DelayGain=.01  enableDrift=off  BetaRef=20*pi/180  KpBeta=1  KpDrift=2  KdDrift=1  KpPsi=6  KOmega=30  tOmega=1  a=l*(1-wd)  b=l*wd  m=m  Cy_f=25266  Cy_r=70933  I=4013  Ksteer=18  theta=45*pi/180  Idl=3  Re=.3  lambda_mu=1  GearInit=0  tShift=.1  pdlVec=[0.1 0.4 0.5 0.9]  upShftTbl=[-1 12.9375 26.4375 39.9375 51.18749999999999 62.4375 72.84375 83.25;-1 16.3125 29.8125 43.3125 54.5624 65.8125 76.78125 87.75;-1 19.6875 33.1875 46.68749999999999 57.9375 69.1875 80.71875 92.25;-1 33 52.5 77.25 100.5 138.75 161.875 185]  dwnShftTbl=[-1 12.9375 26.4375 39.9375 51.18749999999999 62.4375 72.84375 83.25;-1 16.3125 29.8125 43.3125 54.5624 65.8125 76.78125 87.75;-1 19.6875 33.1875 46.68749999999999 57.9375 69.1875 80.71875 92.25;-1 33 52.5 77.25 100.5 138.75 161.875 185]  tClutch=.5  tRev=.5  tPark=120  UpGearVec="[0  1  2  3  4  5  6  7]"  DownGearVec="[1  2  3  4  5  6  7  8]"  aMode=2
  Scope : Scope  NumInputPorts=2
      settings: ActiveDisplayYMinimum=-0.12499999999999997  ActiveDisplayYMaximum=1.125  DataLoggingVariableName=ScopeData9
  Terminator : Terminator
  Terminator1 : Terminator
  Vector Concatenate : Concatenate  NumInputs=3
  km/h 2 m/s : Gain  Gain=1/3.6
  vref - v : Scope  NumInputPorts=2
      settings: ActiveDisplayYMinimum=4.4067398826196023  ActiveDisplayYMaximum=13.304982145555307  DataLoggingVariableName=ScopeData15
  DecelCmd : Outport
  AccelCmd : Outport  Port=2
  wires:
  VehFdbk/1 -> Bus Selector1/1
  km/h 2 m/s/1 -> vref - v/1, Predictive Driver/1
  Constant/1 -> km/h 2 m/s/1
  Constant1/1 -> Predictive Driver/2
  Constant2/1 -> Predictive Driver/3
  Constant3/1 -> Predictive Driver/4
  Predictive Driver/3 -> Scope/1, AccelCmd/1
  Predictive Driver/4 -> Scope/2, DecelCmd/1
  Predictive Driver/2 -> Terminator/1
  Predictive Driver/1 -> Terminator1/1
  Vector Concatenate/1 -> Predictive Driver/6
  Bus Selector1/1 -> vref - v/2, Predictive Driver/5  "<xdot>"
  Bus Selector1/5 -> Predictive Driver/7  "<r>"
  Bus Selector1/2 -> Vector Concatenate/1  "<X>"
  Bus Selector1/3 -> Vector Concatenate/2  "<Y>"
  Bus Selector1/4 -> Vector Concatenate/3  "<psi>"

== system vehicle_cornering_aero_model/Tire/Dual ==
  Fzin : Inport
  VehFdbk : Inport  Port=2
  Dual Fz : Subsystem
  Dual V : Subsystem
  VehVel : Outport  VectorParamsAs1DForOutWhenUnconnected=off
  Fz : Outport  Port=2  VectorParamsAs1DForOutWhenUnconnected=off
  wires:
  Dual V/1(Out1) -> VehVel/1
  VehFdbk/1 -> Dual Fz/1(VehFdbk), Dual V/1(In1)
  Dual Fz/1(Out1) -> Fz/1
  Fzin/1 -> Dual Fz/2(Fzin)

== system vehicle_cornering_aero_model/Tire/Environment ==
  Bus Creator2 : BusCreator  Inputs=2
  Constant1 : Constant  Value=0
  Constant2 : Constant  Value=0
  Constant3 : Constant  Value=ones(1,4)
  Constant6 : Constant  Value=0
  Ground Feedback : Subsystem  Variant=on  VariantControlMode=label  LabelModeActiveChoice=0
  Vector Concatenate1 : Concatenate  NumInputs=3
  Env : Outport  VectorParamsAs1DForOutWhenUnconnected=off
  wires:
  Ground Feedback/1(Ground) -> Bus Creator2/2  "Gnd"
  Vector Concatenate1/1 -> Bus Creator2/1  "Wind"
  Constant2/1 -> Vector Concatenate1/2  "Y"
  Bus Creator2/1 -> Env/1
  Constant6/1 -> Vector Concatenate1/3  "Z"
  Constant1/1 -> Vector Concatenate1/1  "X"
  Constant3/1 -> Ground Feedback/1(Friction)

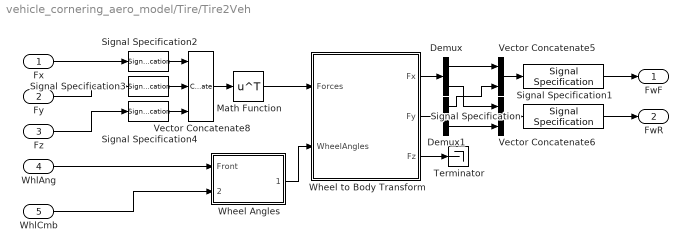
== system vehicle_cornering_aero_model/Tire/Tire2Veh ==
  Fx : Inport
  Fy : Inport  Port=2
  Fz : Inport  Port=3
  WhlAng : Inport  Port=4
  WhlCmb : Inport  Port=5
  Demux : Demux  Outputs=[2,2]
  Demux1 : Demux  Outputs=[2,2]
  Math Function : Math  Operator=transpose  SignedPower=on
  Signal Specification : SignalSpecification  Unit=N
  Signal Specification1 : SignalSpecification  Unit=N
  Signal Specification2 : SignalSpecification  Dimensions=4
  Signal Specification3 : SignalSpecification  Dimensions=4
  Signal Specification4 : SignalSpecification  Dimensions=4
  Terminator : Terminator
  Vector Concatenate5 : Concatenate  Mode=Multidimensional array  ConcatenateDimension=2
  Vector Concatenate6 : Concatenate  Mode=Multidimensional array  ConcatenateDimension=2
  Vector Concatenate8 : Concatenate  NumInputs=3  Mode=Multidimensional array  ConcatenateDimension=2
  Wheel Angles : Subsystem
  Wheel to Body Transform : Subsystem
  FwF : Outport
  FwR : Outport  Port=2
  wires:
  Wheel Angles/1(Vehicle) -> Wheel to Body Transform/2(WheelAngles)
  Vector Concatenate5/1 -> Signal Specification1/1
  Demux/1 -> Vector Concatenate5/1
  Vector Concatenate8/1 -> Math Function/1
  Signal Specification1/1 -> FwF/1
  Wheel to Body Transform/1(Fx) -> Demux/1
  Vector Concatenate6/1 -> Signal Specification/1
  Signal Specification4/1 -> Vector Concatenate8/3
  Demux1/2 -> Vector Concatenate6/2
  Wheel to Body Transform/2(Fy) -> Demux1/1
  Fy/1 -> Signal Specification3/1
  Math Function/1 -> Wheel to Body Transform/1(Forces)
  Wheel to Body Transform/3(Fz) -> Terminator/1
  Demux/2 -> Vector Concatenate6/1
  Signal Specification3/1 -> Vector Concatenate8/2
  Signal Specification2/1 -> Vector Concatenate8/1
  Demux1/1 -> Vector Concatenate5/2
  WhlAng/1 -> Wheel Angles/1(Front)
  Fx/1 -> Signal Specification2/1
  Fz/1 -> Signal Specification4/1
  Signal Specification/1 -> FwR/1
  WhlCmb/1 -> Wheel Angles/2(Camber)

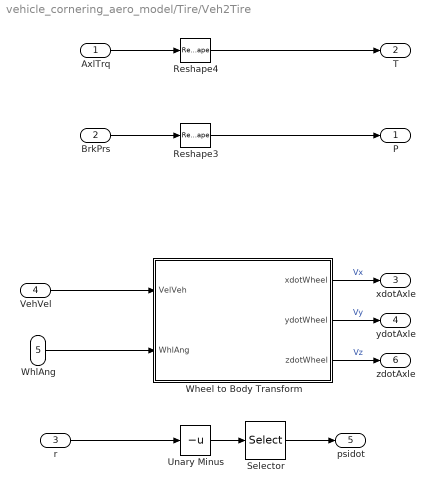
== system vehicle_cornering_aero_model/Tire/Veh2Tire ==
  AxlTrq : Inport
  BrkPrs : Inport  Port=2
  r : Inport  Port=3
  VehVel : Inport  Port=4
  WhlAng : Inport  Port=5
  Reshape3 : Reshape
  Reshape4 : Reshape
  Selector : Selector  InputPortWidth=1  IndexOptions=Index vector (dialog)  Indices=[1 1 1 1]  OutputSizes=1
  Unary Minus : UnaryMinus
  Wheel to Body Transform : Subsystem
  P : Outport  PortDimensions=4  VectorParamsAs1DForOutWhenUnconnected=off
  T : Outport  Port=2  VectorParamsAs1DForOutWhenUnconnected=off
  xdotAxle : Outport  Port=3  PortDimensions=4  VectorParamsAs1DForOutWhenUnconnected=off
  ydotAxle : Outport  Port=4  PortDimensions=4  VectorParamsAs1DForOutWhenUnconnected=off
  psidot : Outport  Port=5  PortDimensions=4  VectorParamsAs1DForOutWhenUnconnected=off
  zdotAxle : Outport  Port=6  VectorParamsAs1DForOutWhenUnconnected=off
  wires:
  BrkPrs/1 -> Reshape3/1
  AxlTrq/1 -> Reshape4/1
  Wheel to Body Transform/1(xdotWheel) -> xdotAxle/1  "Vx"
  Wheel to Body Transform/2(ydotWheel) -> ydotAxle/1  "Vy"
  r/1 -> Unary Minus/1
  Reshape4/1 -> T/1
  VehVel/1 -> Wheel to Body Transform/1(VelVeh)
  Wheel to Body Transform/3(zdotWheel) -> zdotAxle/1  "Vz"
  Unary Minus/1 -> Selector/1
  Reshape3/1 -> P/1
  WhlAng/1 -> Wheel to Body Transform/2(WhlAng)
  Selector/1 -> psidot/1

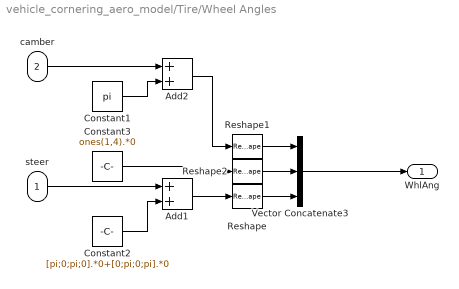
== system vehicle_cornering_aero_model/Tire/Wheel Angles ==
  steer : Inport
  camber : Inport  Port=2
  Add1 : Sum
  Add2 : Sum
  Constant1 : Constant  Value=pi
  Constant2 : Constant  Value=[pi;0;pi;0].*0+[0;pi;0;pi].*0
  Constant3 : Constant  Value=ones(1,4).*0
  Reshape : Reshape  OutputDimensionality=Row vector (2-D)
  Reshape1 : Reshape  OutputDimensionality=Row vector (2-D)
  Reshape2 : Reshape  OutputDimensionality=Row vector (2-D)
  Vector Concatenate3 : Concatenate  NumInputs=3  Mode=Multidimensional array
  WhlAng : Outport  VectorParamsAs1DForOutWhenUnconnected=off
  wires:
  Constant1/1 -> Add2/2
  Add2/1 -> Reshape1/1
  Add1/1 -> Reshape/1
  Reshape2/1 -> Vector Concatenate3/2
  Reshape1/1 -> Vector Concatenate3/1
  Constant3/1 -> Reshape2/1
  camber/1 -> Add2/1
  steer/1 -> Add1/1
  Reshape/1 -> Vector Concatenate3/3
  Vector Concatenate3/1 -> WhlAng/1
  Constant2/1 -> Add1/2

== system vehicle_cornering_aero_model/Tire/scale factors with friction ==
  lamda_mu_x : Inport
  lamda_mu_y : Inport  Port=2
  0 : Constant  Value=[zeros(1,numWheels)]  VectorParams1D=off
  Reshape : Reshape  OutputDimensionality=Row vector (2-D)  OutputDimensions=[1,numWheels]
  Reshape1 : Reshape  OutputDimensionality=Row vector (2-D)  OutputDimensions=[1,numWheels]
  Signal Specification3 : SignalSpecification  Unit=1
  Vector Concatenate : Concatenate  NumInputs=5  Mode=Multidimensional array
  ones : Constant  Value=[ones(23,numWheels)]  VectorParams1D=off
  ones2 : Constant  Value=ones(1,numWheels)  VectorParams1D=off
  lambdas : Outport  Unit=1  VectorParamsAs1DForOutWhenUnconnected=off
  wires:
  lamda_mu_y/1 -> Reshape1/1
  lamda_mu_x/1 -> Reshape/1
  ones2/1 -> Vector Concatenate/1  "lambda_Fz0"
  Vector Concatenate/1 -> Signal Specification3/1
  ones/1 -> Vector Concatenate/5
  0/1 -> Vector Concatenate/4  "lamda_mu_V"
  Reshape1/1 -> Vector Concatenate/3
  Reshape/1 -> Vector Concatenate/2
  Signal Specification3/1 -> lambdas/1

== system vehicle_cornering_aero_model/Tire/Dual/Dual Fz ==
  VehFdbk : Inport
  Fzin : Inport  Port=2
  Add : Sum
  Bus Selector6 : BusSelector  OutputSignals=BdyFrm.Forces.Tires.FrntTires.Lft.Fz,BdyFrm.Forces.Tires.FrntTires.Rght.Fz,BdyFrm.Forces.Tires.RearTires.Lft.Fz,BdyFrm.Forces.Tires.RearTires.Rght.Fz
  Cont LPF : autolibutils/Cont LPF  wc=100*2*pi  AbsoluteTolerance=auto  aMode=2
  Saturation : Saturate  UpperLimit=10e3  LowerLimit=100  ZeroCross=off
  Scope : Scope  NumInputPorts=4
      settings: ActiveDisplayYMinimum=447.595362214918  ActiveDisplayYMaximum=977.316787792114  DataLoggingVariableName=ScopeData6
  Unsprung Mass : Constant  Value="[5 5  5 5].*9.81"
  Out1 : Outport  VectorParamsAs1DForOutWhenUnconnected=off
  wires:
  Saturation/1 -> Cont LPF/1
  Cont LPF/1 -> Add/1
  Fzin/1 -> Saturation/1
  Add/1 -> Out1/1
  Unsprung Mass/1 -> Add/2
  VehFdbk/1 -> Bus Selector6/1
  Bus Selector6/1 -> Scope/1  "<Fz>"
  Bus Selector6/2 -> Scope/2  "<Fz>"
  Bus Selector6/3 -> Scope/3  "<Fz>"
  Bus Selector6/4 -> Scope/4  "<Fz>"

== system vehicle_cornering_aero_model/Tire/Dual/Dual V ==
  In1 : Inport
  Bus Selector1 : BusSelector  OutputSignals=BdyFrm.FrntAxl.Lft.Vel.xdot,BdyFrm.FrntAxl.Lft.Vel.ydot,BdyFrm.FrntAxl.Lft.Vel.zdot  OutputAsBus=on
  Bus Selector2 : BusSelector  OutputSignals=BdyFrm.FrntAxl.Rght.Vel.xdot,BdyFrm.FrntAxl.Rght.Vel.ydot,BdyFrm.FrntAxl.Rght.Vel.zdot  OutputAsBus=on
  Bus Selector4 : BusSelector  OutputSignals=BdyFrm.RearAxl.Lft.Vel.xdot,BdyFrm.RearAxl.Lft.Vel.ydot,BdyFrm.RearAxl.Lft.Vel.zdot  OutputAsBus=on
  Bus Selector5 : BusSelector  OutputSignals=BdyFrm.RearAxl.Rght.Vel.xdot,BdyFrm.RearAxl.Rght.Vel.ydot,BdyFrm.RearAxl.Rght.Vel.zdot  OutputAsBus=on
  Bus to Vector{5..8} (4 alike) : BusToVector
  Vector Concatenate2 : Concatenate  NumInputs=4  Mode=Multidimensional array  ConcatenateDimension=2
  Out1 : Outport  VectorParamsAs1DForOutWhenUnconnected=off
  wires:
  Bus to Vector6/1 -> Vector Concatenate2/2
  Bus Selector2/1 -> Bus to Vector6/1
  Bus to Vector8/1 -> Vector Concatenate2/4
  Bus Selector4/1 -> Bus to Vector7/1
  Bus to Vector5/1 -> Vector Concatenate2/1
  Bus Selector1/1 -> Bus to Vector5/1
  Bus Selector5/1 -> Bus to Vector8/1
  Bus to Vector7/1 -> Vector Concatenate2/3
  Vector Concatenate2/1 -> Out1/1
  In1/1 -> Bus Selector1/1, Bus Selector2/1, Bus Selector4/1, Bus Selector5/1

== system vehicle_cornering_aero_model/Tire/Environment/Ground Feedback ==
  note: 1) Add Subsystem or Model blocks as valid variant choices.
      | 2) You cannot connect blocks at this level. At simulation, connectivity is automatically
      | determined, based on the active variant and port name matching.
  Friction : Inport
  Constant : Subsystem  VariantControl=0
  Ground : Outport  VectorParamsAs1DForOutWhenUnconnected=off

== system vehicle_cornering_aero_model/Tire/Tire2Veh/Wheel Angles ==
  Front : Inport
  Camber : Inport  Port=2
  Constant : Constant  Value=zeros(4,1)
  Reshape : Reshape  OutputDimensionality=Row vector (2-D)
  Reshape1 : Reshape  OutputDimensionality=Row vector (2-D)
  Reshape2 : Reshape  OutputDimensionality=Row vector (2-D)
  Vector Concatenate3 : Concatenate  NumInputs=3  Mode=Multidimensional array
  Vehicle : Outport  VectorParamsAs1DForOutWhenUnconnected=off
  wires:
  Reshape/1 -> Vector Concatenate3/3
  Reshape2/1 -> Vector Concatenate3/2
  Vector Concatenate3/1 -> Vehicle/1
  Reshape1/1 -> Vector Concatenate3/1
  Front/1 -> Reshape/1
  Camber/1 -> Reshape1/1
  Constant/1 -> Reshape2/1

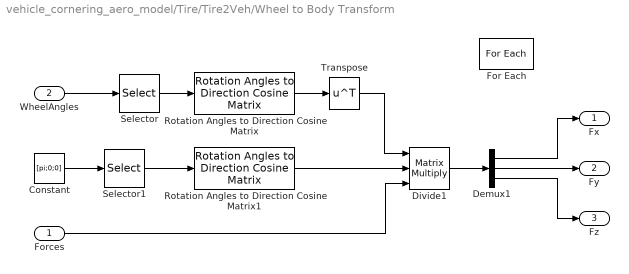
== system vehicle_cornering_aero_model/Tire/Tire2Veh/Wheel to Body Transform ==
  Forces : Inport  PortDimensions=[3,1]  Partition=on  PartitionDimension=2  PartitionWidth=1  PartitionOffset=0
  WheelAngles : Inport  Port=2  Partition=on  PartitionDimension=2  PartitionWidth=1  PartitionOffset=0
  Constant : Constant  Value=[pi;0;0]
  Demux1 : Demux  Outputs=3
  Divide1 : Product  Inputs=***  Multiplication=Matrix(*)
  For Each : ForEach  DisableCoverage=on
  Rotation Angles to Direction Cosine Matrix : sharedtransform/Rotation Angles to Direction Cosine Matrix  rotationOrder=ZYX  aMode=2
  Rotation Angles to Direction Cosine Matrix1 : sharedtransform/Rotation Angles to Direction Cosine Matrix  rotationOrder=ZYX  aMode=2
  Selector : Selector  InputPortWidth=3  IndexOptions=Index vector (dialog)  Indices=[3 2 1]  OutputSizes=1
  Selector1 : Selector  InputPortWidth=3  IndexOptions=Index vector (dialog)  Indices=[3 2 1]  OutputSizes=1
  Transpose : Math  Operator=transpose
  Fx : Outport  ConcatenationDimension=1  VectorParamsAs1DForOutWhenUnconnected=off
  Fy : Outport  Port=2  ConcatenationDimension=1  VectorParamsAs1DForOutWhenUnconnected=off
  Fz : Outport  Port=3  ConcatenationDimension=1  VectorParamsAs1DForOutWhenUnconnected=off
  wires:
  Demux1/1 -> Fx/1
  Demux1/2 -> Fy/1
  Demux1/3 -> Fz/1
  Rotation Angles to Direction Cosine Matrix/1 -> Transpose/1
  Forces/1 -> Divide1/3
  WheelAngles/1 -> Selector/1
  Selector/1 -> Rotation Angles to Direction Cosine Matrix/1
  Rotation Angles to Direction Cosine Matrix1/1 -> Divide1/2
  Divide1/1 -> Demux1/1
  Selector1/1 -> Rotation Angles to Direction Cosine Matrix1/1
  Constant/1 -> Selector1/1
  Transpose/1 -> Divide1/1

== system vehicle_cornering_aero_model/Tire/Veh2Tire/Wheel to Body Transform ==
  VelVeh : Inport  Partition=on  PartitionDimension=2  PartitionWidth=1  PartitionOffset=0
  WhlAng : Inport  Port=2  Partition=on  PartitionDimension=2  PartitionWidth=1  PartitionOffset=0
  Demux1 : Demux  Outputs=3
  Divide1 : Product  Inputs=**  Multiplication=Matrix(*)
  For Each : ForEach  DisableCoverage=on
  Rotation Angles to Direction Cosine Matrix : sharedtransform/Rotation Angles to Direction Cosine Matrix  rotationOrder=ZYX  aMode=2
  Selector : Selector  InputPortWidth=3  IndexOptions=Index vector (dialog)  Indices=[3 2 1]  OutputSizes=1
  xdotWheel : Outport  ConcatenationDimension=1  VectorParamsAs1DForOutWhenUnconnected=off
  ydotWheel : Outport  Port=2  ConcatenationDimension=1  VectorParamsAs1DForOutWhenUnconnected=off
  zdotWheel : Outport  Port=3  ConcatenationDimension=1  VectorParamsAs1DForOutWhenUnconnected=off
  wires:
  Divide1/1 -> Demux1/1
  Demux1/1 -> xdotWheel/1
  Demux1/2 -> ydotWheel/1
  Demux1/3 -> zdotWheel/1
  Rotation Angles to Direction Cosine Matrix/1 -> Divide1/1
  VelVeh/1 -> Divide1/2
  WhlAng/1 -> Selector/1
  Selector/1 -> Rotation Angles to Direction Cosine Matrix/1

== system vehicle_cornering_aero_model/Tire/Environment/Ground Feedback/Constant ==
  Friction : Inport
  Bus Creator : BusCreator  Inputs=4
  Bus Creator2 : BusCreator  Inputs=4
  Bus Creator3 : BusCreator  Inputs=2
  Constant1 : Constant  Value=zeros(4,1)
  Demux : Demux
  Demux1 : Demux
  Signal Specification : SignalSpecification  Unit=m
  Signal Specification1 : SignalSpecification  Unit=1
  Ground : Outport  VectorParamsAs1DForOutWhenUnconnected=off
  wires:
  Bus Creator3/1 -> Ground/1
  Signal Specification1/1 -> Demux1/1
  Friction/1 -> Signal Specification1/1
  Bus Creator2/1 -> Bus Creator3/2  "mu"
  Demux1/2 -> Bus Creator2/2  "mu_FR"
  Demux1/1 -> Bus Creator2/1  "mu_FL"
  Demux1/4 -> Bus Creator2/4  "mu_RR"
  Demux1/3 -> Bus Creator2/3  "mu_RL"
  Bus Creator/1 -> Bus Creator3/1  "z"
  Demux/2 -> Bus Creator/2  "G_FR_z"
  Demux/3 -> Bus Creator/3  "G_RL_z"
  Demux/1 -> Bus Creator/1  "G_FL_z"
  Demux/4 -> Bus Creator/4  "G_RR_z"
  Signal Specification/1 -> Demux/1
  Constant1/1 -> Signal Specification/1

== matlab function vehicle_cornering_aero_model/scope/MATLAB Function1 ==
  data: FyFL input; MB output; FyFR input; FyRL input; FyRR input; Fyf output; Fyr output; Fy output
function [MB, Fyf, Fyr, Fy] = fcn(FyFL, FyFR, FyRL, FyRR)

Fyf = FyFL + FyFR;

Fyr = FyRL + FyRR;

MB = Fyr*100/(Fyf+Fyr);

Fy = Fyf + Fyr;

== matlab function vehicle_cornering_aero_model/scope/MATLAB Function ==
  data: vx input; SAFL output; vy input; r input; SAFR output; WHfl input; WHfr input; WHrl input; WHrr input; l input; wd input; SARL output; SARR output; Tf input; Tr input
function [SAFL, SAFR, SARL, SARR] = fcn(vx, vy, r, WHfl, WHfr, WHrl, WHrr, l, wd,Tf, Tr)

SAFL = -(vy+r*l*(1-wd))/(vx-r*Tf/2)-WHfl;

SAFR = -(vy+r*l*(1-wd))/(vx+r*Tf/2)-WHfr;

SARL = -(vy-r*l*wd)/(vx-r*Tr/2)-WHrl;

SARR = -(vy-r*l*wd)/(vx+r*Tr/2)-WHrr;

== matlab function vehicle_cornering_aero_model/Powertrain/Motor speed limit ==
  data: spd input; MtrSpd output; spdlim input
function MtrSpd = fcn(spd, spdlim)

if spd<spdlim
    MtrSpd = spd;
else
    MtrSpd = spdlim;
end

== matlab function vehicle_cornering_aero_model/Powertrain/Acc Curve ==
  data: Acc input; MtrTrq output; Trqmax input
function MtrTrq = fcn(Acc, Trqmax)

MtrTrq = Trqmax*Acc;

== matlab function vehicle_cornering_aero_model/Powertrain/Torque Determination ==
  data: power input; MtrSpd input; Trqmax output
function Trqmax  = fcn(power, MtrSpd)

Trq = power/(MtrSpd*2*pi/60);

if Trq <= maxTrq
    Trqmax = Trq;
else
    Trqmax = maxTrq;
end

== matlab function vehicle_cornering_aero_model/ロール剛性/荷重移動量計算 ==
  data: dwf output; phi input; ay input; dwr output; Kpf parameter; Kpr parameter; m parameter; l parameter; wd parameter; RCf parameter; RCr parameter; track parameter
%ロール角を計算
function [dwf, dwr]  = fcn(phi, ay, Kpf, Kpr, m, l, wd, RCf, RCr, track)

%ロール運動の方程式からロール角とロール速度を微分方程式を計算して算出する
%自動車の運動と制御第2版のP.176参照

df = track(1,1);
dr = track(1,2);
%荷重移動量計算
%Fr
dwf = (Kpf*phi+(ay*9.806*m*(1-wd)*RCf)/l)/df;

%Rr
dwr = (Kpr*phi+(ay*9.806*m*wd*RCr)/l)/dr;

== matlab function vehicle_cornering_aero_model/ロール剛性/各輪荷重計算 ==
  data: dwf input; FzFL output; dwr input; FzFR output; FzRL output; FzRR output; m parameter; wd parameter
function [FzFL, FzFR, FzRL, FzRR] = fcn(dwf, dwr, m, wd)

FzFL = 0.5*m*wd*9.806 + dwf;
FzFR = 0.5*m*wd*9.806 - dwf;
FzRL = 0.5*m*(1-wd)*9.806 + dwr;
FzRR = 0.5*m*(1-wd)*9.806 - dwr;
